simulink model "a2"  (R2021b)
settings: Solver=VariableStepAuto  StartTime=0.0  StopTime=180  RelTol=1e-3
settings Model: Creator=郭义月  LastModifiedBy=郭义月

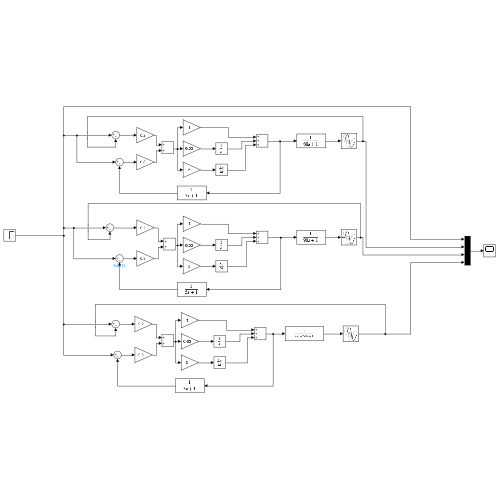
[thumbnail: Simulink's stored preview of the top-level diagram]
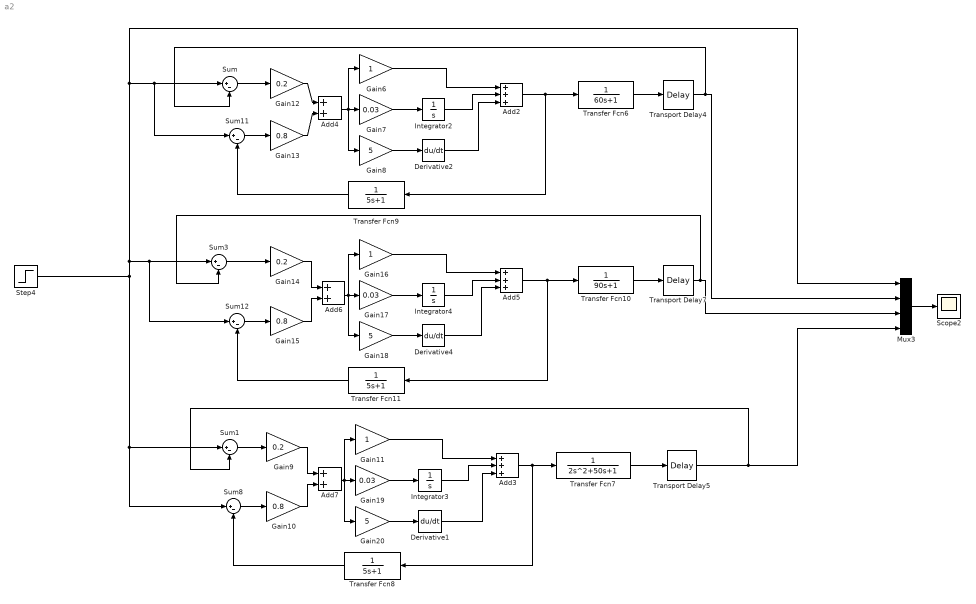
== system a2 ==
  Add2 : Sum  Inputs=+++
  Add3 : Sum  Inputs=+++
  Add4 : Sum
  Add5 : Sum  Inputs=+++
  Add6 : Sum
  Add7 : Sum
  Derivative1 : Derivative
  Derivative2 : Derivative
  Derivative4 : Derivative
  Gain10 : Gain  Gain=0.8
  Gain11 : Gain
  Gain12 : Gain  Gain=0.2
  Gain13 : Gain  Gain=0.8
  Gain14 : Gain  Gain=0.2
  Gain15 : Gain  Gain=0.8
  Gain16 : Gain
  Gain17 : Gain  Gain=0.03
  Gain18 : Gain  Gain=5
  Gain19 : Gain  Gain=0.03
  Gain20 : Gain  Gain=5
  Gain6 : Gain
  Gain7 : Gain  Gain=0.03
  Gain8 : Gain  Gain=5
  Gain9 : Gain  Gain=0.2
  Integrator2 : Integrator
  Integrator3 : Integrator
  Integrator4 : Integrator
  Mux3 : Mux
  Scope2 : Scope
  Step4 : Step  SampleTime=0
  Sum{,1,3,8,11..12} (6 alike) : Sum  Inputs=|+-
  Transfer Fcn10 : TransferFcn  Denominator=[90 1]
  Transfer Fcn11 : TransferFcn  Denominator=[5 1]
  Transfer Fcn6 : TransferFcn  Denominator=[60 1]
  Transfer Fcn7 : TransferFcn  Denominator=[2 50 1]
  Transfer Fcn8 : TransferFcn  Denominator=[5 1]
  Transfer Fcn9 : TransferFcn  Denominator=[5 1]
  Transport Delay4 : TransportDelay  DelayTime=30
  Transport Delay5 : TransportDelay  DelayTime=30
  Transport Delay7 : TransportDelay  DelayTime=30
  wires:
  Sum8/1 -> Gain10/1
  Transfer Fcn7/1 -> Transport Delay5/1
  Transport Delay4/1 -> Sum/2, Mux3/2
  Sum12/1 -> Gain15/1
  Derivative4/1 -> Add5/3
  Transfer Fcn11/1 -> Sum12/2
  Integrator2/1 -> Add2/2
  Gain9/1 -> Add7/1
  Gain6/1 -> Add2/1
  Gain10/1 -> Add7/2
  Derivative2/1 -> Add2/3
  Transfer Fcn10/1 -> Transport Delay7/1
  Gain20/1 -> Derivative1/1
  Transfer Fcn6/1 -> Transport Delay4/1
  Integrator3/1 -> Add3/2
  Mux3/1 -> Scope2/1
  Step4/1 -> Sum8/1, Sum1/1, Sum12/1, Sum3/1, Sum11/1, Sum/1, Mux3/1
  Transfer Fcn9/1 -> Sum11/2
  Gain12/1 -> Add4/1
  Gain18/1 -> Derivative4/1
  Gain7/1 -> Integrator2/1
  Gain19/1 -> Integrator3/1
  Transfer Fcn8/1 -> Sum8/2
  Gain8/1 -> Derivative2/1
  Add7/1 -> Gain20/1, Gain11/1, Gain19/1
  Add3/1 -> Transfer Fcn8/1, Transfer Fcn7/1
  Gain13/1 -> Add4/2
  Sum11/1 -> Gain13/1
  Add6/1 -> Gain18/1, Gain16/1, Gain17/1
  Transport Delay7/1 -> Sum3/2, Mux3/3
  Gain14/1 -> Add6/1
  Integrator4/1 -> Add5/2
  Gain16/1 -> Add5/1
  Add4/1 -> Gain8/1, Gain6/1, Gain7/1
  Sum/1 -> Gain12/1
  Gain17/1 -> Integrator4/1
  Gain15/1 -> Add6/2
  Transport Delay5/1 -> Sum1/2, Mux3/4
  Gain11/1 -> Add3/1
  Add2/1 -> Transfer Fcn9/1, Transfer Fcn6/1
  Add5/1 -> Transfer Fcn11/1, Transfer Fcn10/1
  Derivative1/1 -> Add3/3
  Sum3/1 -> Gain14/1
  Sum1/1 -> Gain9/1
